simulink model "controller"  (R2023b)
settings: Solver=ode1  StartTime=0.0  StopTime=inf  FixedStep=0.02  RelTol=1e-3  EnableMultiTasking=on
model workspace (MAT data in the model file):
  K = [0.0327 40.9616 0.2758 -296.3349 2.2732]
  Ki = 100
undefined symbols (not defined in the file or in its folder): DiscIntNeverNeededParam
libraries: simulink x1
settings Model: Creator=danie  LastModifiedBy=danie
settings SolverCC: AutoInsertRateTranBlk=on  InsertRTBMode=Always
settings OptimizationCC: DefaultParameterBehavior=Inlined  EnhancedBackFolding=on  PassReuseOutputArgsAs=Individual arguments  ZeroExternalMemoryAtStartup=off  ZeroInternalMemoryAtStartup=off  MaxStackSize=64  OptimizeBlockOrder=speed  DifferentSizesBufferReuse=on  OptimizationCustomize=off  EfficientTunableParamExpr=on
settings DebuggingCC: ParameterTunabilityLossMsg=error
settings HardwareCC: ProdBitPerPointer=32  ProdBitPerSizeT=32  ProdBitPerPtrDiffT=32  ProdLargestAtomicInteger=Long  ProdLargestAtomicFloat=Double  ProdWordSize=32  ProdHWDeviceType=ARM Compatible->ARM Cortex-M
settings SFSimCC: MATLABDynamicMemAlloc=off
settings RTWCC: Description=Embedded Coder  SystemTargetFile=ert.tlc  GenCodeOnly=on  TemplateMakefile=ert_default_tmf  Toolchain=GNU Tools for ARM Embedded Processors
settings CodeAppCC: ForceParamTrailComments=on  IgnoreCustomStorageClasses=off  OperatorAnnotations=on  SimulinkDataObjDesc=on  SFDataObjDesc=on  InsertBlockDesc=on
settings ERTTargetCC: GenerateSampleERTMain=on  InlinedParameterPlacement=NonHierarchical  ERTCustomFileTemplate=example_file_process.tlc

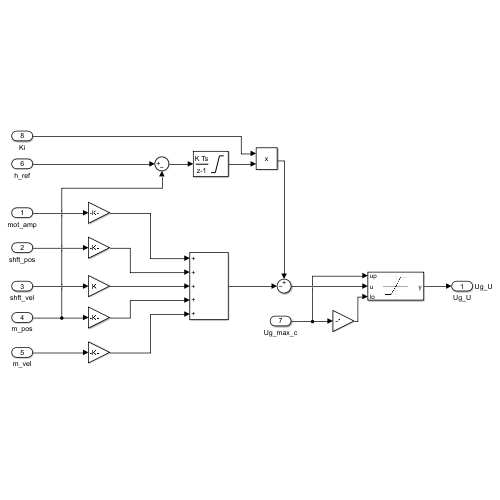
[thumbnail: Simulink's stored preview of the top-level diagram]
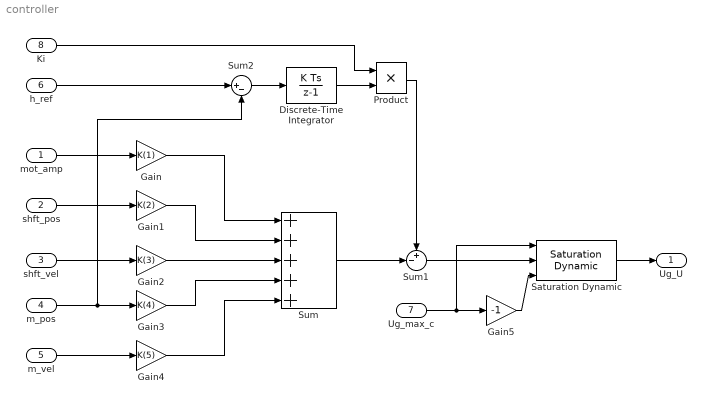
== system controller ==
  mot_amp : Inport
  shft_pos : Inport  Port=2
  shft_vel : Inport  Port=3
  m_pos : Inport  Port=4
  m_vel : Inport  Port=5
  h_ref : Inport  Port=6
  Ug_max_c : Inport  Port=7
  Ki : Inport  Port=8
  Discrete-Time Integrator : DiscreteIntegrator  SampleTime=0.02  LimitOutput=on  UpperSaturationLimit=200  LowerSaturationLimit=-200  ICPrevOutput=DiscIntNeverNeededParam  ICPrevScaledInput=DiscIntNeverNeededParam
  Gain : Gain  Gain=K(1)
  Gain1 : Gain  Gain=K(2)
  Gain2 : Gain  Gain=K(3)
  Gain3 : Gain  Gain=K(4)
  Gain4 : Gain  Gain=K(5)
  Gain5 : Gain  Gain=-1
  Product : Product
  Saturation Dynamic : simulink/Discontinuities/Saturation Dynamic  OutMin=[]  OutMax=[]  OutDataTypeStr=Inherit: Same as second input  OutDataType=fixdt(1, 16)  OutScaling=2^-10  DoSatur=off
  Sum : Sum  Inputs=+++++
  Sum1 : Sum  Inputs=+-|
  Sum2 : Sum  Inputs=|+-
  Ug_U : Outport  SignalName=Ug_U
  wires:
  Gain/1 -> Sum/1
  Gain1/1 -> Sum/2
  Gain2/1 -> Sum/3
  Gain4/1 -> Sum/5
  Gain3/1 -> Sum/4
  mot_amp/1 -> Gain/1
  shft_pos/1 -> Gain1/1
  shft_vel/1 -> Gain2/1
  m_pos/1 -> Sum2/2, Gain3/1
  m_vel/1 -> Gain4/1
  Sum/1 -> Sum1/2
  Sum1/1 -> Saturation Dynamic/2
  Saturation Dynamic/1 -> Ug_U/1
  Ug_max_c/1 -> Gain5/1, Saturation Dynamic/1
  Discrete-Time Integrator/1 -> Product/2
  h_ref/1 -> Sum2/1
  Sum2/1 -> Discrete-Time Integrator/1
  Product/1 -> Sum1/1
  Ki/1 -> Product/1
  Gain5/1 -> Saturation Dynamic/3
